simulink model "inp_blocks"  (R2024b)
settings: Solver=VariableStepAuto  StartTime=0.0  StopTime=10.0  RelTol=1e-3
libraries: simulink x3
settings Model: Creator=FREED  LastModifiedBy=acer

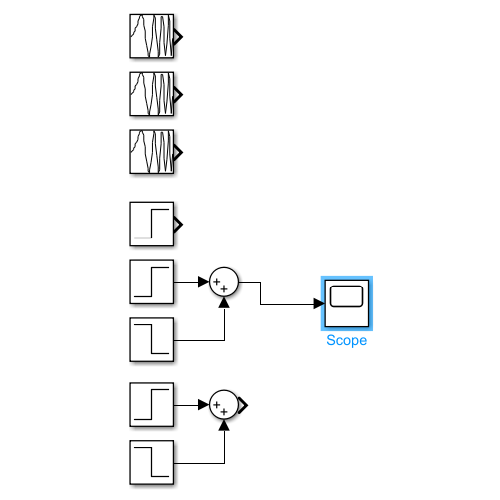
[thumbnail: Simulink's stored preview of the top-level diagram]
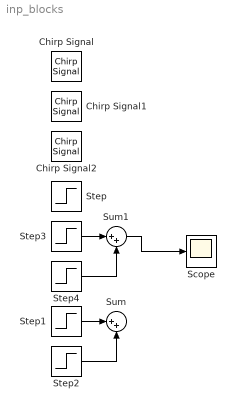
== system inp_blocks ==
  Chirp Signal : simulink/Sources/Chirp Signal  f1=0.1  T=10  f2=1
  Chirp Signal1 : simulink/Sources/Chirp Signal  f1=1  T=10  f2=5
  Chirp Signal2 : simulink/Sources/Chirp Signal  f1=5  T=10  f2=1  VectorParams1D=off
  Scope : Scope
  Step : Step  Time=5  Before=6  After=12  SampleTime=0
  Step1 : Step  Time=5  Before=6  After=12  SampleTime=0
  Step2 : Step  Time=8  After=-24  SampleTime=0
  Step3 : Step  Time=5  Before=6  After=12  SampleTime=0
  Step4 : Step  Time=8  After=-6  SampleTime=0
  Sum : Sum  Inputs=|++
  Sum1 : Sum  Inputs=|++
  wires:
  Step2/1 -> Sum/2
  Step1/1 -> Sum/1
  Step3/1 -> Sum1/1
  Step4/1 -> Sum1/2
  Sum1/1 -> Scope/1
